simulink model "Accelerometer"  (R2019b)
settings: Solver=FixedStepAuto  StartTime=0.0  StopTime=10  FixedStep=1e-5  RelTol=1e-3
InitFcn:
  | clear
  | close all
  | clc
  | 
  | %------------------------optical fiber given constants
  | Y = 7*10^10; % Young modulus [n/m^2]
  | Y = 7.54*10^10; % Young modulus [n/m^2]
  | L = 4.5*10^-2; % length [m]
  | D = 125*10^-6; % diameter [m]
  | A = pi*(D/2)^2; % area [m^2]
  | 
  | m = 22.23*10^-3 ; % mass [kg]
  | 
  | k = Y*A/L; % spring stiffness [kg/s^2]
  | k = 4*k; % equivalent spring for 4 optical fibers
  | w0 = sqrt(k/m) ; % [Hz]
  | f0 = w0/(2*pi)
  | %y = b/m; % damping factor in [1/s]
  | 
  | y = 1.521; % damping factor from Antune, 2009. [1/s]
  | b = y*m; % [kg/s]
  | 
  | 
  | %------------------------transfer functions
  | accel = tf( [1], [1 y k/m])
  | ramp = tf([1], [1 0])
StopFcn:
  | set(groot,'defaultAxesTickLabelInterpreter','latex')
  | set(groot,'defaultLegendInterpreter','latex')
  | figure('Units','centimeter','Position',[0 0 10 7],'PaperPositionMode','auto')
  | plot(out.output.Time,out.output.Data,'color',[.3 .3 .3])
  | ylabel('Position [m]','interpreter','latex')
  | xlabel('Time [s]','interpreter','latex')
  | 
  | belize =[41/255 128/255 185/255]
  | hold on
  | yyaxis right
  | plot(out.output.Time,out.input.Data,'linewidth',1.5,'color',belize)
  | xlim([out.output.Time(1)-0.5 out.output.Time(end)])
  | ylabel('Acceleration input [m/s$^2$]','interpreter','latex')
  | set(gca,'YColor','k')
  | ylim([-0.5 1.5])
  | 
  | 
  | %% Alan script
  | t =out.output.Time;
  | vs = out.output.Data;
  | 
  | vs=vs-mean(vs);
  | vf=abs(2*fft(vs)/length(vs));
  | %amplitudes
  | f=(0:length(vs)-1)./(max(t)-min(t));
  | %frequ^encias
  | vf=vf(1:round(length(vs)/2));
  | f=f(1:round(length(vs)/2));
  | %frequenciadepico
  | [~,p]=max(vf);
  | %encontrar minimos laterais(limites para calculo da media)
  | p1=p(1);
  | p2=p(1);
  | aux=0.5*max(vf);
  | while vf(p1)>aux&&p1>1%lado esquerdo
  | 	p1=p1-1;
  | end
  | 
  | while vf(p2)>aux&&p2<length(f)%lado direito
  | 	p2=p2+1;
  | end
  | %encontrar frequencia central
  | fs=trapz(f(p1:p2),f(p1:p2).*vf(p1:p2))/trapz(f(p1:p2),vf(p1:p2));
  | %valores de pico
  | [~,p1]=findpeaks(vs,'MinPeakHeight',0);
  | [~,p2]=findpeaks(-vs,'MinPeakHeight',0);
  | while length(p1)>length(p2)
  | 	p1=p1(1:end-1);
  | end
  | while length(p1)<length(p2)
  | 	p2=p2(1:end-1);
  | end
  | vpp=vs(p1)-vs(p2);
  | tpp=t(p1);
  | %identificar decaimento
  | pol=polyfit(tpp,log(vpp),1);
  | as=real(pol(1));
  | 
  | %% show results
  | display(['Input damping factor [1/s]= ',num2str(y)])
  | display(['System resonance [Hz]= ',num2str(w0/(2*pi))])
  | legend(['$f_0$ = ', num2str(mean(fs)),'[Hz]',10,'$\Gamma$ = ',num2str(-as*2),'[1/s]'],'Acceleration','interpreter','latex')
settings Model: Creator=Stinky  LastModifiedBy=Stinky

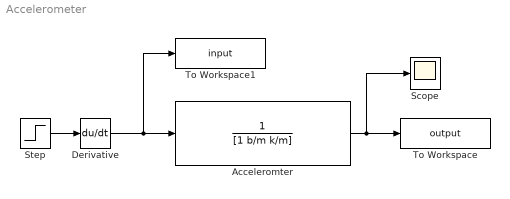
== system Accelerometer ==
  Acceleromter : TransferFcn  Denominator=[1 b/m k/m]
  Derivative : Derivative
  Scope : Scope
  Step : Step  Time=0.1  SampleTime=0
  To Workspace : ToWorkspace  VariableName=output  SaveFormat=Timeseries  SampleTime=-1
  To Workspace1 : ToWorkspace  VariableName=input  SaveFormat=Timeseries  SampleTime=-1
  wires:
  Acceleromter/1 -> Scope/1, To Workspace/1
  Step/1 -> Derivative/1
  Derivative/1 -> To Workspace1/1, Acceleromter/1
